simulink model "sumador"  (R2022a)
settings: Solver=VariableStepAuto  StartTime=0.0  StopTime=10.0  RelTol=1e-3
settings Model: Creator=Estudiantes  LastModifiedBy=Estudiantes

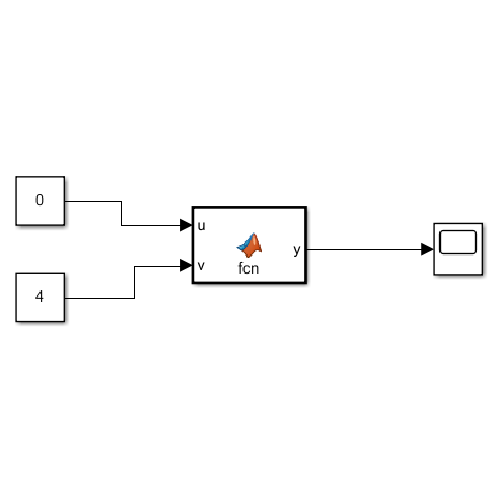
[thumbnail: Simulink's stored preview of the top-level diagram]
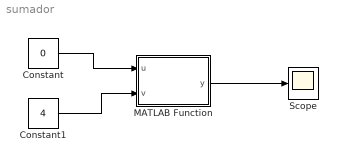
== system sumador ==
  Constant : Constant  Value=0
  Constant1 : Constant  Value=4
  MATLAB Function : MATLAB Function  TreatAsAtomicUnit=on
  Scope : Scope
  wires:
  Constant/1 -> MATLAB Function/1(u)
  Constant1/1 -> MATLAB Function/2(v)
  MATLAB Function/1(y) -> Scope/1

== matlab function sumador/MATLAB Function ==
  data: u input; y output; v input
function y = fcn(u,v)

s=0;

for c = 1:v
    s=s+u;
end
y=s;
